simulink model "control_az4_1"  (R2019b)
settings: Solver=FixedStepAuto  StartTime=0.0  StopTime=0.5  FixedStep=1e-5  RelTol=1e-3
settings Model: Creator=SamRayaneh  LastModifiedBy=SamRayaneh

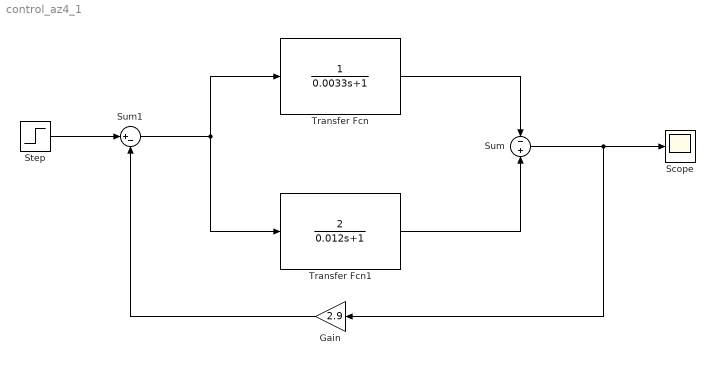
== system control_az4_1 ==
  Gain : Gain  Gain=2.9
  Scope : Scope
  Step : Step  Time=0.1  SampleTime=0
  Sum : Sum  Inputs=-+
  Sum1 : Sum  Inputs=|+-
  Transfer Fcn : TransferFcn  Denominator=[0.0033 1]
  Transfer Fcn1 : TransferFcn  Numerator=[2]  Denominator=[0.012 1]
  wires:
  Transfer Fcn/1 -> Sum/1
  Transfer Fcn1/1 -> Sum/2
  Step/1 -> Sum1/1
  Sum1/1 -> Transfer Fcn/1, Transfer Fcn1/1
  Sum/1 -> Gain/1, Scope/1
  Gain/1 -> Sum1/2
